simulink model "submarine"  (R2024a)
settings: Solver=FixedStepAuto  StartTime=0.0  StopTime=inf  FixedStep=0.1  RelTol=1e-3
settings Model: Creator=nicol  LastModifiedBy=nicol

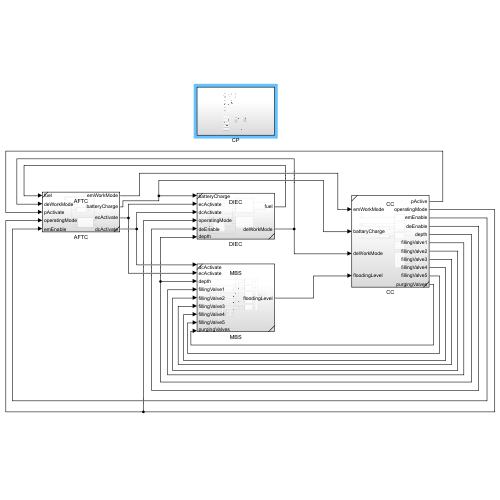
[thumbnail: Simulink's stored preview of the top-level diagram]
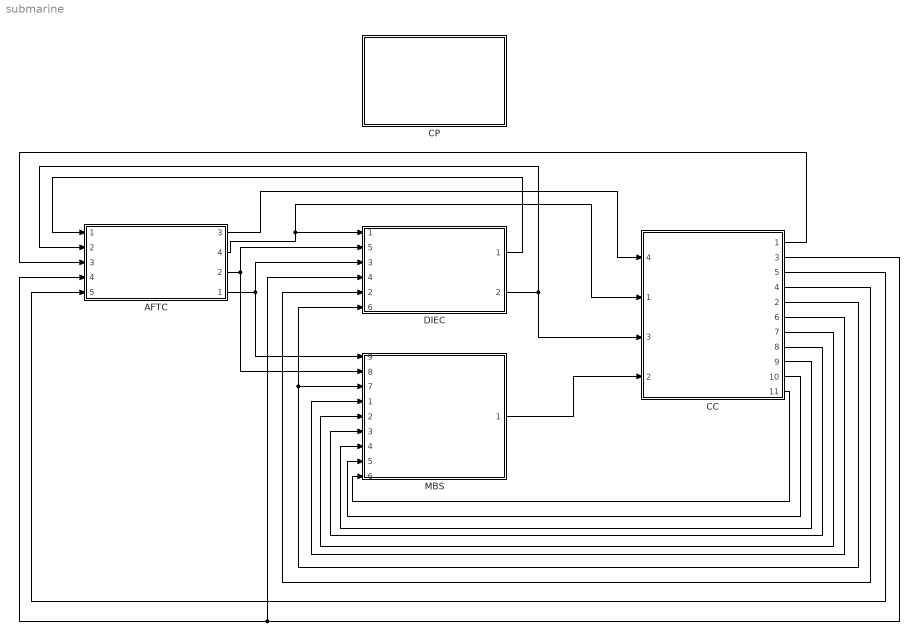
== system submarine ==
  AFTC : Subsystem  ReferencedSubsystem=AFTC
      settings: PortSchema="{\"entries\":[{\"content\":{\"sides\":[{\"content\":{\"connectorIds\":[\"In1\",\"In2\",\"In3\",\"In4\",\"In5\"]},\"type\":\"ConnectorPlacement.EquallySpacedRectSide\",\"uuid\":\"5dd9e4a6-9723-4f84-b8ea-64015c68d220\"},{\"content\":{\"connectorIds\":[\"Out3\",\"Out4\",\"Out2\",\"Out1\"],\"side\":\"RIGHT\"},\"type\":\"ConnectorPlacement.EquallySpacedRectSide\",\"uuid\":\"489282da-3ac6-4763-8bc7-59e61995c82c\"},{\"content\":{\"side\":\"TOP\"},\"type\":\"ConnectorPlacement.EquallySpacedRectSide\",\"uuid\":\"0c55a21b-bab5-4126-bb05-3f198729d59d\"}]},\"type\":\"ConnectorPlacement.EquallySpacedConnector\",\"uuid\":\"619cc89b-07fc-45e6-bd20-c28f67fe96fc\"}],\"packageUris\":[\"http://schema.mathworks.com/mf0/Connector/R2020b\"],\"version\":\"1.0\"}"
  CC : Subsystem  ReferencedSubsystem=CC
      settings: PortSchema="{\"entries\":[{\"content\":{\"sides\":[{\"content\":{\"connectorIds\":[\"In4\",\"In1\",\"In3\",\"In2\"]},\"type\":\"ConnectorPlacement.EquallySpacedRectSide\",\"uuid\":\"dad31c5b-656f-495e-9d27-1396e330f301\"},{\"content\":{\"connectorIds\":[\"Out1\",\"Out3\",\"Out5\",\"Out4\",\"Out2\",\"Out6\",\"Out7\",\"Out8\",\"Out9\",\"Out10\",\"Out11\"],\"side\":\"RIGHT\"},\"type\":\"ConnectorPlacement.EquallySpacedRectSide\",\"uuid\":\"7cd86499-dcc7-4464-bfee-b19392297322\"},{\"content\":{\"side\":\"TOP\"},\"type\":\"ConnectorPlacement.EquallySpacedRectSide\",\"uuid\":\"e7abb689-a986-4b10-9963-2a1b507f78b8\"}]},\"type\":\"ConnectorPlacement.EquallySpacedConnector\",\"uuid\":\"e7cdd45f-ad78-4470-b804-f2db0f07f6b7\"}],\"packageUris\":[\"http://schema.mathworks.com/mf0/Connector/R2020b\"],\"version\":\"1.0\"}"
  CP : Subsystem
  DIEC : Subsystem  ReferencedSubsystem=DIEC
      settings: PortSchema="{\"entries\":[{\"content\":{\"sides\":[{\"content\":{\"connectorIds\":[\"In1\",\"In5\",\"In3\",\"In4\",\"In2\",\"In6\"]},\"type\":\"ConnectorPlacement.EquallySpacedRectSide\",\"uuid\":\"67395347-15b1-4edd-beb9-db80eb8fe3e8\"},{\"content\":{\"connectorIds\":[\"Out1\",\"Out2\"],\"side\":\"RIGHT\"},\"type\":\"ConnectorPlacement.EquallySpacedRectSide\",\"uuid\":\"4ac8abce-2b52-4275-9a87-52aab28d1303\"},{\"content\":{\"side\":\"TOP\"},\"type\":\"ConnectorPlacement.EquallySpacedRectSide\",\"uuid\":\"4f0b87f4-c2d0-4f91-94fc-e33d93605f55\"}]},\"type\":\"ConnectorPlacement.EquallySpacedConnector\",\"uuid\":\"57701178-ddee-44b7-aa7f-3e8254ce849f\"}],\"packageUris\":[\"http://schema.mathworks.com/mf0/Connector/R2020b\"],\"version\":\"1.0\"}"
  MBS : Subsystem  ReferencedSubsystem=MBS
      settings: PortSchema="{\"entries\":[{\"content\":{\"sides\":[{\"content\":{\"connectorIds\":[\"In9\",\"In8\",\"In7\",\"In1\",\"In2\",\"In3\",\"In4\",\"In5\",\"In6\"]},\"type\":\"ConnectorPlacement.EquallySpacedRectSide\",\"uuid\":\"7719223a-62f2-4610-8bb3-ceefc10589c1\"},{\"content\":{\"connectorIds\":[\"Out1\"],\"side\":\"RIGHT\"},\"type\":\"ConnectorPlacement.EquallySpacedRectSide\",\"uuid\":\"75d7257f-d30d-49e5-a80a-3ba0e31cfda1\"},{\"content\":{\"side\":\"TOP\"},\"type\":\"ConnectorPlacement.EquallySpacedRectSide\",\"uuid\":\"d7e7af29-945e-4e76-8618-c9bd92d8b648\"}]},\"type\":\"ConnectorPlacement.EquallySpacedConnector\",\"uuid\":\"77094e27-0841-4602-9c83-2abd814a6f06\"}],\"packageUris\":[\"http://schema.mathworks.com/mf0/Connector/R2020b\"],\"version\":\"1.0\"}"
  wires:
  AFTC/1 -> DIEC/3, MBS/9
  AFTC/2 -> MBS/8, DIEC/5
  AFTC/3 -> CC/4
  AFTC/4 -> DIEC/1, CC/1
  DIEC/1 -> AFTC/1
  DIEC/2 -> CC/3, AFTC/2
  CC/1 -> AFTC/3
  CC/2 -> DIEC/6, MBS/7
  CC/3 -> AFTC/4, DIEC/4
  CC/4 -> DIEC/2
  CC/5 -> AFTC/5
  CC/11 -> MBS/6
  CC/10 -> MBS/5
  CC/9 -> MBS/4
  CC/8 -> MBS/3
  CC/7 -> MBS/2
  CC/6 -> MBS/1
  MBS/1 -> CC/2

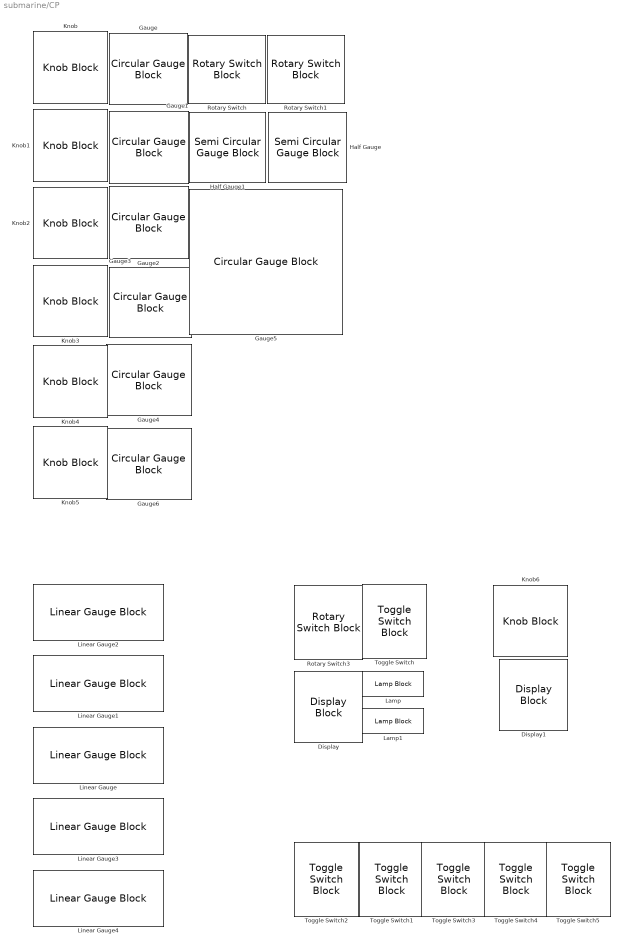
== system submarine/CP ==
  Display : DisplayBlock  LabelPosition=Hide  Transparency=1
  Display1 : DisplayBlock  LabelPosition=Hide  Transparency=1
  Gauge{,1..4,6} (6 alike) : CircularGaugeBlock
  Gauge5 : CircularGaugeBlock  ScaleMax=260
  Half Gauge : SemiCircularGaugeBlock  ScaleMin=-35  ScaleMax=35  ScaleDirection=Counterclockwise
  Half Gauge1 : SemiCircularGaugeBlock  ScaleMin=-40  ScaleMax=40
  Knob{,1..5} (6 alike) : KnobBlock
  Knob6 : KnobBlock  ScaleMin=-35  ScaleMax=35
  Lamp : LampBlock
  Lamp1 : LampBlock
  Linear Gauge : LinearGaugeBlock  ScaleMax=3000
  Linear Gauge1 : LinearGaugeBlock  ScaleMax=50000
  Linear Gauge2 : LinearGaugeBlock  ScaleMax=3000
  Linear Gauge3 : LinearGaugeBlock  ScaleMax=360
  Linear Gauge4 : LinearGaugeBlock  ScaleMax=240
  Rotary Switch : RotarySwitchBlock
      settings: Values={{'Down', 'Const', 'Up'}, [-1 0 1]}
  Rotary Switch1 : RotarySwitchBlock
      settings: Values={{'Down', 'Const', 'Up'}, [-1 0 1]}
  Rotary Switch3 : RotarySwitchBlock
      settings: Values={{'TFSA', 'FSA', 'AF', 'SF', 'TSF', 'BES', 'CtB', 'TSB', 'SB', 'MB', 'TMCB'}, [0 1 2 3 4 5 6 7 8 9 10]}
  Toggle Switch{,1..5} (6 alike) : ToggleSwitchBlock
